simulink model "IndirectMRAC"  (R2019b)
settings: Solver=VariableStepAuto  StartTime=0.0  StopTime=100  RelTol=1e-3
libraries: simulink x1
settings Model: Creator=chint  LastModifiedBy=chint

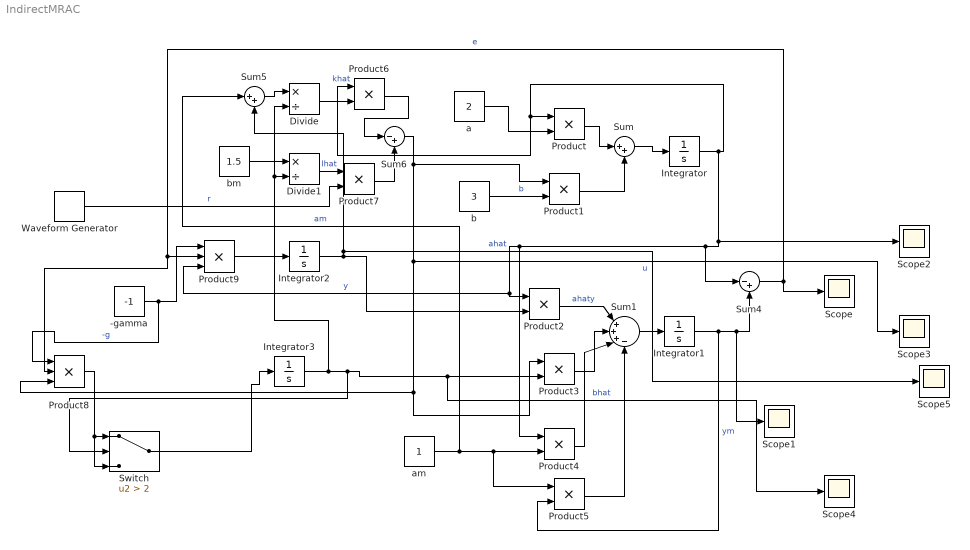
== system IndirectMRAC ==
  -gamma : Constant  Value=-1
  Divide : Product  Inputs=*/
  Divide1 : Product  Inputs=*/
  Integrator : Integrator  InitialCondition=1
  Integrator1 : Integrator  InitialCondition=1
  Integrator2 : Integrator  InitialCondition=10
  Integrator3 : Integrator  InitialCondition=-10
  Product{,1..7} (8 alike) : Product
  Product8 : Product  Inputs=3
  Product9 : Product  Inputs=3
  Scope{,1..5} (6 alike) : Scope
  Sum : Sum  Inputs=|++
  Sum1 : Sum  Inputs=|+++-
  Sum4 : Sum  Inputs=|-+
  Sum5 : Sum  Inputs=|++
  Sum6 : Sum  Inputs=|-+
  Switch : Switch  Criteria=u2 > Threshold  Threshold=2
  Waveform Generator : simulink/Sources/Waveform Generator  OutMin=[]  OutMax=[]  OutDataTypeStr=double  SelectedSignal=1  Signals=sin(5,6,7)+sin(6,4,8)  BlockNames=MultiportSwitch_4389fe67d3434a5  SampleTime=0.1
      settings: SourceProductName=Simulink
  a : Constant  Value=2
  am : Constant
  b : Constant  Value=3
  bm : Constant  Value=1.5
  wires:
  Integrator/1 -> Scope2/1, Sum4/1, Product9/3, Product2/1, Product4/1, Product6/2, Product/1  "y"
  a/1 -> Product/2
  b/1 -> Product1/2  "b"
  Product/1 -> Sum/1
  Product1/1 -> Sum/2
  Sum/1 -> Integrator/1
  Product3/1 -> Sum1/2
  Product2/1 -> Sum1/1  "ahaty"
  Integrator2/1 -> Product2/2, Sum5/2, Scope5/1  "ahat"
  Integrator3/1 -> Divide1/2, Divide/2, Switch/2, Scope4/1, Product3/2  "bhat"
  Sum1/1 -> Integrator1/1
  Sum6/1 -> Product1/1, Product8/3, Product3/1, Scope3/1  "u"
  Product4/1 -> Sum1/3
  am/1 -> Sum5/1, Product5/1, Product4/2  "am"
  Product5/1 -> Sum1/4
  Integrator1/1 -> Scope1/1, Sum4/2, Product5/2  "ym"
  Product8/1 -> Switch/3, Switch/1
  Product9/1 -> Integrator2/1
  -gamma/1 -> Product9/1, Product8/1  "-g"
  Sum4/1 -> Product8/2, Product9/2, Scope/1  "e"
  bm/1 -> Divide1/1
  Sum5/1 -> Divide/1
  Divide/1 -> Product6/1  "khat"
  Divide1/1 -> Product7/1  "lhat"
  Waveform Generator/1 -> Product7/2  "r"
  Product6/1 -> Sum6/1
  Product7/1 -> Sum6/2
  Switch/1 -> Integrator3/1
